simulink model "testTD"  (R2018a)
settings: Solver=VariableStepAuto  StartTime=0.0  StopTime=81  RelTol=1e-3
settings Model: Creator=Ducted Fan  LastModifiedBy=Ducted Fan

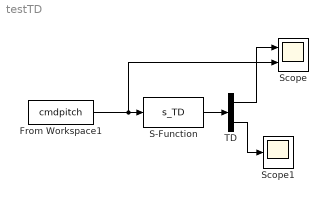
== system testTD ==
  From Workspace1 : FromWorkspace  VariableName=cmdpitch  SampleTime=0
  S-Function : S-Function  FunctionName=s_TD  SFunctionDeploymentMode=off  EnableBusSupport=off
  Scope : Scope  NumInputPorts=2
  Scope1 : Scope
  TD : Demux  Outputs=2
  wires:
  From Workspace1/1 -> Scope/2, S-Function/1
  S-Function/1 -> TD/1
  TD/1 -> Scope/1
  TD/2 -> Scope1/1
